simulink library "target_gen_logic_lib"  (R2018b)
settings: Solver=VariableStepAuto  StartTime=0.0  StopTime=10.0  RelTol=1e-3
libraries: simulink x2
settings Model: Creator=Taylor  LastModifiedBy=Taylor

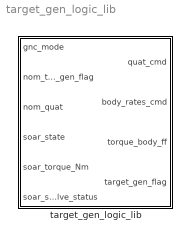
== system target_gen_logic_lib ==
  target_gen_logic_lib : Subsystem

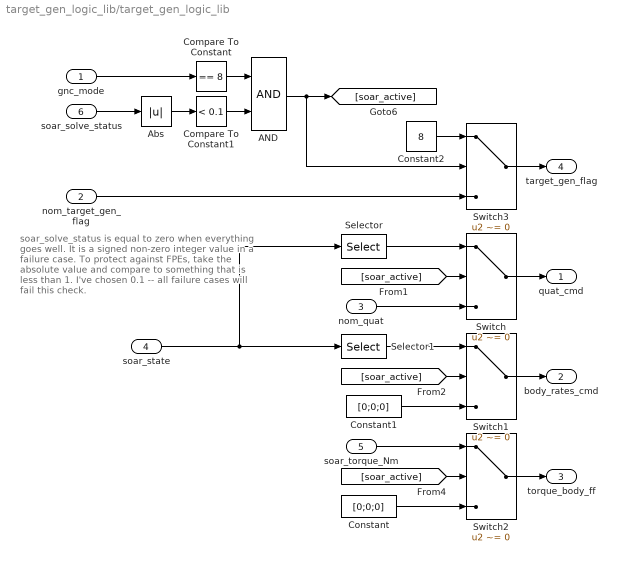
== system target_gen_logic_lib/target_gen_logic_lib ==
  note: soar_solve_status is equal to zero
      | when everything goes well. It is a signed
      | non-zero integer value in a failure case.
      | To protect against FPEs, take the absolute
      | value and compare to something that is
      | less than 1. I've chosen 0.1 -- all failure cases
      | will fail this check.
  gnc_mode : Inport
  nom_target_gen_flag : Inport  Port=2
  nom_quat : Inport  Port=3
  soar_state : Inport  Port=4
  soar_torque_Nm : Inport  Port=5
  soar_solve_status : Inport  Port=6
  AND : Logic  AllPortsSameDT=off  OutDataTypeStr=boolean
  Abs : Abs
  Compare To Constant : simulink/Logic and Bit Operations/Compare To Constant  relop===  const=8  OutDataTypeStr=boolean
  Compare To Constant1 : simulink/Logic and Bit Operations/Compare To Constant  relop=<  const=0.1  OutDataTypeStr=boolean
  Constant : Constant  Value=[0;0;0]  OutDataTypeStr=double
  Constant1 : Constant  Value=[0;0;0]  OutDataTypeStr=double
  Constant2 : Constant  Value=8  OutDataTypeStr=uint8
  Selector : Selector  InputPortWidth=10  IndexOptions=Index vector (dialog)  Indices=[1 2 3 4]  OutputSizes=1
  Selector1 : Selector  InputPortWidth=10  IndexOptions=Index vector (dialog)  Indices=[5 6 7]  OutputSizes=1
  Switch : Switch  Criteria=u2 ~= 0  OutDataTypeStr=double  InputSameDT=on
  Switch1 : Switch  Criteria=u2 ~= 0  OutDataTypeStr=double  InputSameDT=on
  Switch2 : Switch  Criteria=u2 ~= 0  OutDataTypeStr=double  InputSameDT=on
  Switch3 : Switch  Criteria=u2 ~= 0  OutDataTypeStr=uint8  InputSameDT=on
  quat_cmd : Outport
  body_rates_cmd : Outport  Port=2
  torque_body_ff : Outport  Port=3
  target_gen_flag : Outport  Port=4
  wires:
  Switch1/1 -> body_rates_cmd/1
  [soar_active] -> Switch/2
  Switch/1 -> quat_cmd/1
  Switch2/1 -> torque_body_ff/1
  nom_quat/1 -> Switch/3
  [soar_active] -> Switch2/2
  [soar_active] -> Switch1/2
  gnc_mode/1 -> Compare To Constant/1
  AND/1 -> Switch3/2, [soar_active]
  soar_state/1 -> Selector/1, Selector1/1
  Compare To Constant/1 -> AND/1
  soar_solve_status/1 -> Abs/1
  soar_torque_Nm/1 -> Switch2/1
  Constant/1 -> Switch2/3
  Constant1/1 -> Switch1/3
  Selector1/1 -> Switch1/1
  Selector/1 -> Switch/1
  Compare To Constant1/1 -> AND/2
  Abs/1 -> Compare To Constant1/1
  Switch3/1 -> target_gen_flag/1
  nom_target_gen_flag/1 -> Switch3/3
  Constant2/1 -> Switch3/1
